simulink model "HandDryer_Controller"  (R2024b)
settings: Solver=FixedStepDiscrete  StartTime=0.0  StopTime=10.0  FixedStep=0.1  RelTol=1e-3  EnableMultiTasking=on
settings Model: Creator=58  LastModifiedBy=58
settings SolverCC: AlgebraicLoopSolver=TrustRegion  AutoInsertRateTranBlk=on
settings DataIOCC: LimitDataPoints=on
settings OptimizationCC: LifeSpan=inf
settings DebuggingCC: UnconnectedInputMsg=warning  UnconnectedOutputMsg=warning  UnconnectedLineMsg=warning  AllowSymbolicDim=off  SFUnexpectedBacktrackingDiag=warning  SFNoUnconditionalDefaultTransitionDiag=warning  SFExecutionAtInitializationDiag=none  ArithmeticOperatorsInVariantConditions=warning
settings ModelReferenceCC: EnableRefExpFcnMdlSchedulingChecks=on
settings SFSimCC: SimUseLocalCustomCode=off  CustomCodeUndefinedFunction=UseInterfaceOnly
settings RTWCC: RTWUseLocalCustomCode=off  GPUComputeCapability=3.5  DLArmComputeVersion=19.05
settings CodeAppCC: StateflowObjectComments=on
settings GRTTargetCC: TargetLangStandard=C89/C90 (ANSI)
settings ConfigComp: CovMetricSettings=dw  CovSaveCumulativeToWorkspaceVar=on  CovSaveSingleToWorkspaceVar=on  CovExternalEMLEnable=off  CovSFcnEnable=off

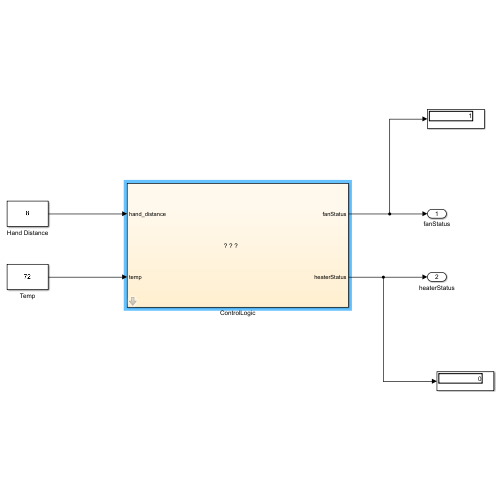
[thumbnail: Simulink's stored preview of the top-level diagram]
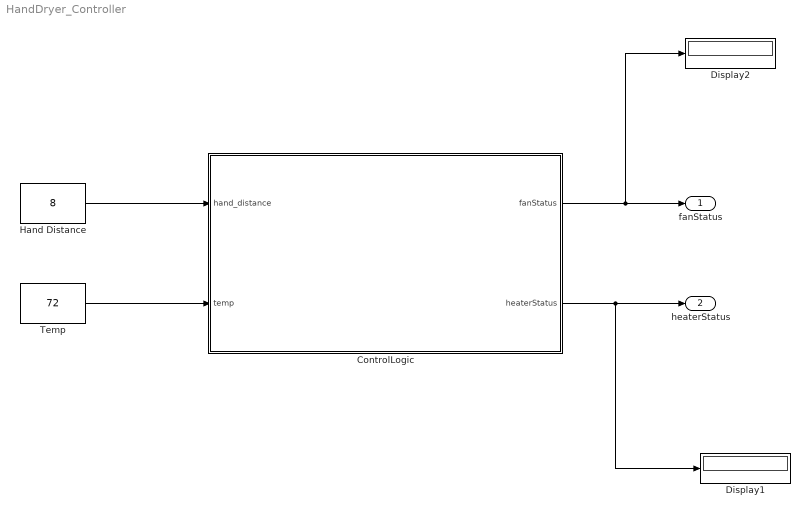
== system HandDryer_Controller ==
  ControlLogic : Stateflow chart  TreatAsAtomicUnit=on
  Display1 : Display
  Display2 : Display
  Hand Distance : Constant  Value=8
  Temp : Constant  Value=72
  fanStatus : Outport
  heaterStatus : Outport  Port=2
  wires:
  Hand Distance/1 -> ControlLogic/1(hand_distance)
  Temp/1 -> ControlLogic/2(temp)
  ControlLogic/2(heaterStatus) -> heaterStatus/1, Display1/1
  ControlLogic/1(fanStatus) -> Display2/1, fanStatus/1

== stateflow chart HandDryer_Controller/ControlLogic ==
  state Active
    state lowTemp
      en:
      fanStatus=true;
      heaterStatus=true;
    state highTemp
      en:
      fanStatus=true;
      heaterStatus=false;
    (default) -> (junction 18)
    (junction 18) -> lowTemp [order 1] : [temp<65]
    (junction 18) -> highTemp [order 2]
    highTemp -> lowTemp : [temp<65]
    lowTemp -> highTemp : [temp>070]
  state Idle
    en:
    fanStatus = false ;
    heaterStatus = false ;
  state waiteState
  state waiteState2
  (default) -> Idle
  waiteState -> Active [order 1] : after(1,sec)
  Idle -> waiteState : [hand_distance<10]
  waiteState -> Idle [order 2] : [hand_distance>=10]
  Active -> waiteState2 [order 1] : [hand_distance>15]
  waiteState2 -> Idle [order 2] : after(3,sec)
  waiteState2 -> Active [order 1] : [hand_distance<=15]
  Active -> Idle [order 2] : after(60,sec)
  data: hand_distance input double; fanStatus output boolean; heaterStatus output boolean; temp input double
